simulink model "simulink_Lab5"  (R2022a)
settings: Solver=FixedStepAuto  StartTime=0.0  StopTime=10.0  FixedStep=1e-3  RelTol=1e-3
values from neighbouring files (symbols this model uses):
  K = 5    [sim_lab5_sc.m]
  Taw = 2    [sim_lab5_sc.m]
settings Model: Creator=bebawy  LastModifiedBy=bebawy
settings OptimizationCC: DefaultParameterBehavior=Inlined  UseDivisionForNetSlopeComputation=on  GainParamInheritBuiltInType=on  UseFloatMulNetSlope=on  InlineInvariantSignals=on  EfficientFloat2IntCast=on  LifeSpan=1
settings RTWCC: GenerateReport=on  LaunchReport=on
settings CodeAppCC: ForceParamTrailComments=on
settings GRTTargetCC: CombineSignalStateStructs=on  MatFileLogging=off  SupportVariableSizeSignals=on

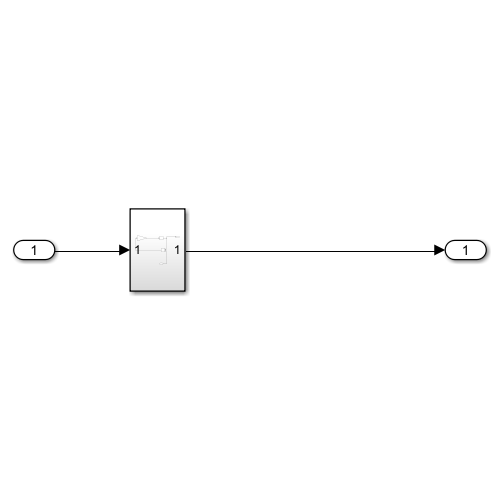
[thumbnail: Simulink's stored preview of the top-level diagram]
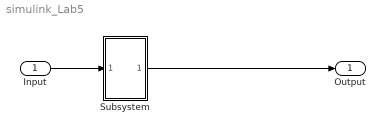
== system simulink_Lab5 ==
  Input : Inport
  Subsystem : Subsystem
  Output : Outport
  wires:
  Input/1 -> Subsystem/1(Input)
  Subsystem/1(Output) -> Output/1

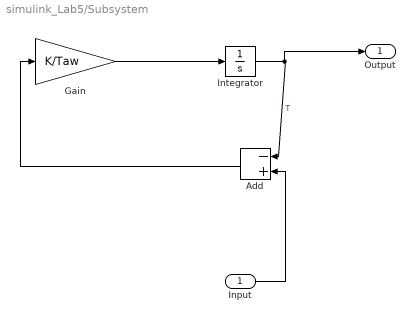
== system simulink_Lab5/Subsystem ==
  Input : Inport
  Add : Sum  Inputs=-+
  Gain : Gain  Gain=K/Taw
  Integrator : Integrator
  Output : Outport
  wires:
  Integrator/1 -> Output/1, Add/1  "T"
  Add/1 -> Gain/1
  Input/1 -> Add/2
  Gain/1 -> Integrator/1
